simulink model "siasun_config_casadi_VS_lsj_sim_16a"  (R2019b)
settings: Solver=FixedStepAuto  StartTime=0.0  StopTime=20  FixedStep=0.001  RelTol=1e-3  EnableMultiTasking=on
undefined symbols (not defined in the file): a1, a2, a3, d1, d4, fc1, fc2, fc3, fc4, fc5, fc6, fv1, fv2, fv3, fv4, fv5, fv6, Ia1, Ia2, Ia3, Ia4, Ia5, Ia6, Ic111, Ic112, Ic113, Ic122, Ic123, Ic133, Ic211, Ic212, Ic213, Ic222, Ic223, Ic233, Ic311, Ic312, Ic313, Ic322, Ic323, Ic333, Ic411, Ic412, Ic413, Ic422, Ic423, Ic433, Ic511, Ic512, Ic513, Ic522, Ic523, Ic533, Ic611, Ic612, Ic613, Ic622, Ic623, Ic633, m1 ... (+26)
libraries: sm_lib x224, nesl_utility x124, simulink x8
(part 1 of 10)
settings Model: Creator=Administrator  LastModifiedBy=admin
settings SolverCC: AlgebraicLoopSolver=LineSearch
settings DataIOCC: ReturnWorkspaceOutputs=off
settings OptimizationCC: LifeSpan=inf
settings DebuggingCC: SFUnexpectedBacktrackingDiag=warning  SFNoUnconditionalDefaultTransitionDiag=warning  ArithmeticOperatorsInVariantConditions=warning
settings SFSimCC: SimUseLocalCustomCode=off  CustomCodeUndefinedFunction=UseInterfaceOnly
settings RTWCC: RTWUseLocalCustomCode=off
settings CodeAppCC: StateflowObjectComments=on
settings GRTTargetCC: TargetLangStandard=C89/C90 (ANSI)
settings ConfigComp: CovMetricSettings=dw  CovSaveCumulativeToWorkspaceVar=on  CovSaveSingleToWorkspaceVar=on  CovExternalEMLEnable=off
settings SimscapeCC: SimscapeNormalizeSystem=off
settings ExplorerConfigSet: InternalSimMechanicsExplorerSettings="<ExplorerConfiguration><canonicalview>default</canonicalview><AnimationSetting><BasePlaybackSpeed>1.0</BasePlaybackSpeed><PlaybackSpeedFactor>1.0</PlaybackSpeedFactor></AnimationSetting><TilePanel><TileInfo><Tiles Columns=\"1\" Count=\"1\" Rows=\"1\"><Column Left=\"2\" Weight=\"1\"/><Column Left=\"307\"/><Row Top=\"2\" Weight=\"1\"/><Row Top=\"464\"/><Tile Height=\"1\" Width=\"1\" X=\"0\" Y=\"0\"/></Tiles></TileInfo><SceneInfo><SceneViewer><BGColor><R>0.60000002384185791</R><G>0.60000002384185791</G><B>0.60000002384185791</B></BGColor><Camera><DoPerspective>off</DoPerspective><Position><X>0.25771122604707614</X><Y>-0.76959052816919193</Y><Z>0.37589669226781303</Z></Position><Center><X>0.25771122604707614</X><Y>0.14257423281669612</Y><Z>0.37589669226781303</Z></Center><Up><X>0</X><Y>-0</Y><Z>1</Z></Up><ViewLimDist>1</ViewLimDist><YLim>0.6801680654881832</YLim><XLim>0.44443652844260978</XLim></Camera></SceneViewer></SceneInfo></TilePanel><MechEditorPanel><Cameras/><GfxPanelCameraMap/></MechEditorPanel></ExplorerConfiguration>"

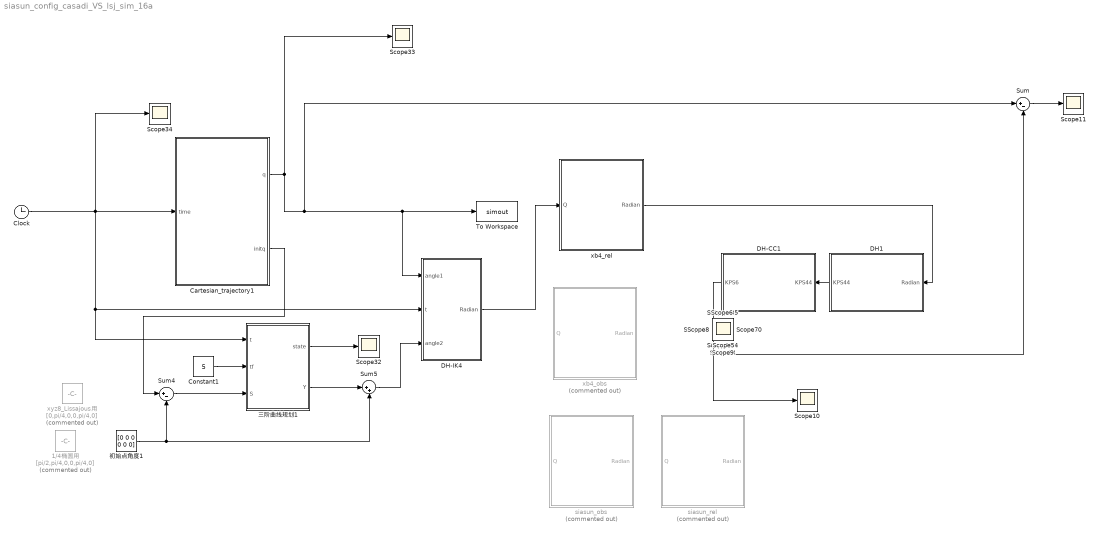
== system siasun_config_casadi_VS_lsj_sim_16a ==
  1/4椭圆用 : Constant  Commented=on  Value=[pi/2,pi/4,0,0,pi/4,0]
  Cartesian_trajectory1 : MATLAB Function  TreatAsAtomicUnit=on
  Clock : Clock
  Constant1 : Constant  Value=5
  DH-CC1 : MATLAB Function  TreatAsAtomicUnit=on
  DH-IK4 : MATLAB Function  TreatAsAtomicUnit=on
  DH1 : MATLAB Function  TreatAsAtomicUnit=on
  Scope{,1..34} (35 alike) : Scope
  Sum : Sum  Inputs=|+-
  Sum4 : Sum  Inputs=|+-
  Sum5 : Sum  Inputs=|++
  To Workspace : ToWorkspace  VariableName=simout  SampleTime=-1
      settings: Save2DSignal=2-D array (concatenate along first dimension)
  siasun_obs : Subsystem  Commented=on
  siasun_rel : Subsystem  Commented=on
  xb4_obs : Subsystem  Commented=on
  xb4_rel : Subsystem
  xyz8_Lissajous用 : Constant  Commented=on  Value=[0,pi/4,0,0,pi/4,0]
  三阶曲线规划1 : Subsystem
  初始点角度1 : Constant  Value=[0 0 0 0 0 0]
  wires:
  DH-IK4/1(Radian) -> xb4_rel/1(Q)
  Cartesian_trajectory1/1(q) -> To Workspace/1, DH-IK4/1(angle1), Sum/1, Scope33/1
  初始点角度1/1 -> Sum5/2, Sum4/2
  Sum4/1 -> 三阶曲线规划1/3(S)
  Constant1/1 -> 三阶曲线规划1/2(tf)
  三阶曲线规划1/1(state) -> Scope32/1
  三阶曲线规划1/2(Y) -> Sum5/1
  Sum5/1 -> DH-IK4/3(angle2)
  Clock/1 -> DH-IK4/2(t), 三阶曲线规划1/1(t), Scope34/1, Cartesian_trajectory1/1(time)
  xb4_rel/1(Radian) -> DH1/1(Radian)
  DH1/1(KPS44) -> DH-CC1/1(KPS44)
  DH-CC1/1(KPS6) -> Sum/2, Scope10/1
  Cartesian_trajectory1/2(initq) -> Sum4/1
  Sum/1 -> Scope11/1

== system siasun_config_casadi_VS_lsj_sim_16a/siasun_obs ==
  Q : Inport
  Discrete Derivative : simulink/Discrete/Discrete Derivative  gainval=1.0  ICPrevScaledInput=0.0  OutMin=[]  OutMax=[]  OutDataType=fixdt(1, 16)  OutScaling=2^-10  DoSatur=off
  Discrete Derivative1 : simulink/Discrete/Discrete Derivative  gainval=1.0  ICPrevScaledInput=0.0  OutMin=[]  OutMax=[]  OutDataType=fixdt(1, 16)  OutScaling=2^-10  DoSatur=off
  Robot : Subsystem
  Scope : Scope
  Scope1 : Scope
  Terminator : Terminator
  Terminator1 : Terminator
  Terminator2 : Terminator
  Radian : Outport
  wires:
  Discrete Derivative1/1 -> Robot/3(qdd), Scope/1
  Discrete Derivative/1 -> Robot/2(qd), Discrete Derivative1/1, Scope1/1
  Q/1 -> Robot/1(q), Discrete Derivative/1
  Robot/4(t) -> Terminator2/1
  Robot/3(b) -> Terminator1/1
  Robot/2(w) -> Terminator/1
  Robot/1(Q) -> Radian/1

== system siasun_config_casadi_VS_lsj_sim_16a/siasun_rel ==
  Q : Inport
  Discrete Derivative : simulink/Discrete/Discrete Derivative  gainval=1.0  ICPrevScaledInput=0.0  OutMin=[]  OutMax=[]  OutDataType=fixdt(1, 16)  OutScaling=2^-10  DoSatur=off
  Discrete Derivative1 : simulink/Discrete/Discrete Derivative  gainval=1.0  ICPrevScaledInput=0.0  OutMin=[]  OutMax=[]  OutDataType=fixdt(1, 16)  OutScaling=2^-10  DoSatur=off
  Robot : Subsystem
  Scope : Scope
  Scope1 : Scope
  Terminator : Terminator
  Terminator1 : Terminator
  Terminator2 : Terminator
  Radian : Outport
  wires:
  Discrete Derivative1/1 -> Robot/3(qdd), Scope/1
  Discrete Derivative/1 -> Robot/2(qd), Discrete Derivative1/1, Scope1/1
  Q/1 -> Robot/1(q), Discrete Derivative/1
  Robot/4(t) -> Terminator2/1
  Robot/3(b) -> Terminator1/1
  Robot/2(w) -> Terminator/1
  Robot/1(Q) -> Radian/1

== system siasun_config_casadi_VS_lsj_sim_16a/xb4_obs ==
  Q : Inport
  Discrete Derivative : simulink/Discrete/Discrete Derivative  gainval=1.0  ICPrevScaledInput=0.0  OutMin=[]  OutMax=[]  OutDataType=fixdt(1, 16)  OutScaling=2^-10  DoSatur=off
  Discrete Derivative1 : simulink/Discrete/Discrete Derivative  gainval=1.0  ICPrevScaledInput=0.0  OutMin=[]  OutMax=[]  OutDataType=fixdt(1, 16)  OutScaling=2^-10  DoSatur=off
  Robot : Subsystem
  Scope : Scope
  Scope1 : Scope
  Terminator : Terminator
  Terminator1 : Terminator
  Terminator2 : Terminator
  Radian : Outport
  wires:
  Discrete Derivative1/1 -> Robot/3(qdd), Scope/1
  Discrete Derivative/1 -> Robot/2(qd), Discrete Derivative1/1, Scope1/1
  Q/1 -> Robot/1(q), Discrete Derivative/1
  Robot/4(t) -> Terminator2/1
  Robot/3(b) -> Terminator1/1
  Robot/2(w) -> Terminator/1
  Robot/1(Q) -> Radian/1

== system siasun_config_casadi_VS_lsj_sim_16a/xb4_rel ==
  Q : Inport
  Discrete Derivative : simulink/Discrete/Discrete Derivative  gainval=1.0  ICPrevScaledInput=0.0  OutMin=[]  OutMax=[]  OutDataType=fixdt(1, 16)  OutScaling=2^-10  DoSatur=off
  Discrete Derivative1 : simulink/Discrete/Discrete Derivative  gainval=1.0  ICPrevScaledInput=0.0  OutMin=[]  OutMax=[]  OutDataType=fixdt(1, 16)  OutScaling=2^-10  DoSatur=off
  Robot : Subsystem
  Scope : Scope
  Scope1 : Scope
  Terminator : Terminator
  Terminator1 : Terminator
  Terminator2 : Terminator
  Radian : Outport
  wires:
  Robot/1(Q) -> Radian/1
  Robot/2(w) -> Terminator/1
  Robot/3(b) -> Terminator1/1
  Robot/4(t) -> Terminator2/1
  Q/1 -> Discrete Derivative/1, Robot/1(q)
  Discrete Derivative/1 -> Scope1/1, Discrete Derivative1/1, Robot/2(qd)
  Discrete Derivative1/1 -> Scope/1, Robot/3(qdd)

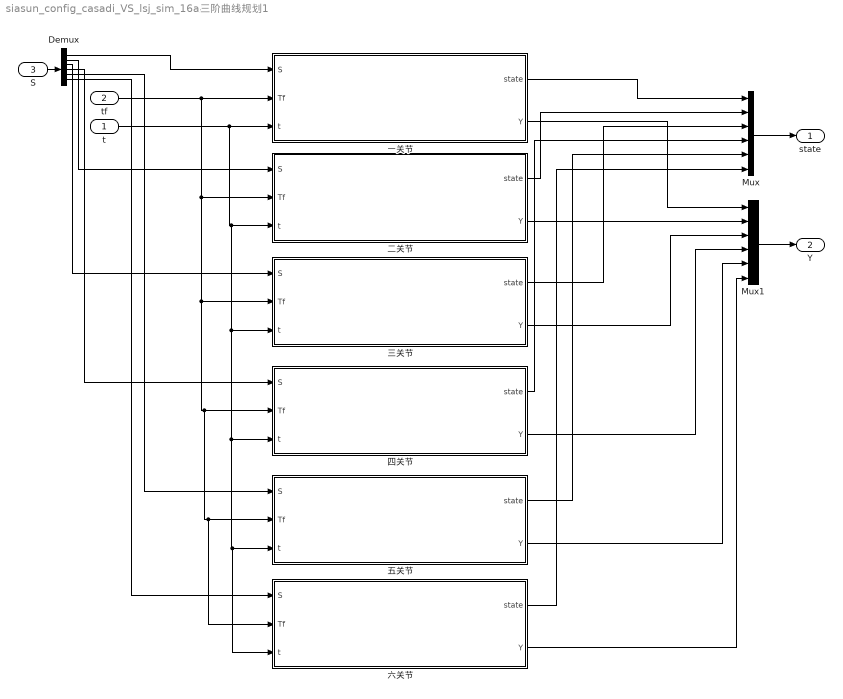
== system siasun_config_casadi_VS_lsj_sim_16a/三阶曲线规划1 ==
  t : Inport
  tf : Inport  Port=2
  S : Inport  Port=3
  Demux : Demux  Outputs=6
  Mux : Mux  Inputs=6
  Mux1 : Mux  Inputs=6
  一关节 : Subsystem
  三关节 : Subsystem
  二关节 : Subsystem
  五关节 : Subsystem
  六关节 : Subsystem
  四关节 : Subsystem
  state : Outport
  Y : Outport  Port=2
  wires:
  一关节/2(Y) -> Mux1/1
  tf/1 -> 六关节/2(Tf), 五关节/2(Tf), 四关节/2(Tf), 三关节/2(Tf), 二关节/2(Tf), 一关节/2(Tf)
  t/1 -> 六关节/3(t), 五关节/3(t), 四关节/3(t), 三关节/3(t), 二关节/3(t), 一关节/3(t)
  一关节/1(state) -> Mux/1
  三关节/1(state) -> Mux/3
  二关节/1(state) -> Mux/2
  四关节/1(state) -> Mux/4
  S/1 -> Demux/1
  Demux/1 -> 一关节/1(S)
  Demux/2 -> 二关节/1(S)
  Demux/3 -> 三关节/1(S)
  Demux/4 -> 四关节/1(S)
  Demux/5 -> 五关节/1(S)
  Demux/6 -> 六关节/1(S)
  Mux1/1 -> Y/1
  二关节/2(Y) -> Mux1/2
  三关节/2(Y) -> Mux1/3
  四关节/2(Y) -> Mux1/4
  五关节/2(Y) -> Mux1/5
  六关节/2(Y) -> Mux1/6
  Mux/1 -> state/1
  五关节/1(state) -> Mux/5
  六关节/1(state) -> Mux/6

== system siasun_config_casadi_VS_lsj_sim_16a/siasun_obs/Robot ==
  q : Inport
  qd : Inport  Port=2
  qdd : Inport  Port=3
  Robot : Subsystem
  Q : Outport
  w : Outport  Port=2
  b : Outport  Port=3
  t : Outport  Port=4
  wires:
  qdd/1 -> Robot/3(qdd)
  qd/1 -> Robot/2(qd)
  q/1 -> Robot/1(q)
  Robot/4(t) -> t/1
  Robot/3(b) -> b/1
  Robot/2(w) -> w/1
  Robot/1(Q) -> Q/1

== system siasun_config_casadi_VS_lsj_sim_16a/siasun_rel/Robot ==
  q : Inport
  qd : Inport  Port=2
  qdd : Inport  Port=3
  Robot : Subsystem
  Q : Outport
  w : Outport  Port=2
  b : Outport  Port=3
  t : Outport  Port=4
  wires:
  qdd/1 -> Robot/3(qdd)
  qd/1 -> Robot/2(qd)
  q/1 -> Robot/1(q)
  Robot/4(t) -> t/1
  Robot/3(b) -> b/1
  Robot/2(w) -> w/1
  Robot/1(Q) -> Q/1

== system siasun_config_casadi_VS_lsj_sim_16a/xb4_obs/Robot ==
  q : Inport
  qd : Inport  Port=2
  qdd : Inport  Port=3
  Robot : Subsystem
  Q : Outport
  w : Outport  Port=2
  b : Outport  Port=3
  t : Outport  Port=4
  wires:
  qdd/1 -> Robot/3(qdd)
  qd/1 -> Robot/2(qd)
  q/1 -> Robot/1(q)
  Robot/4(t) -> t/1
  Robot/3(b) -> b/1
  Robot/2(w) -> w/1
  Robot/1(Q) -> Q/1

== system siasun_config_casadi_VS_lsj_sim_16a/xb4_rel/Robot ==
  q : Inport
  qd : Inport  Port=2
  qdd : Inport  Port=3
  Robot : Subsystem
  Q : Outport
  w : Outport  Port=2
  b : Outport  Port=3
  t : Outport  Port=4
  wires:
  Robot/1(Q) -> Q/1
  Robot/2(w) -> w/1
  Robot/3(b) -> b/1
  Robot/4(t) -> t/1
  q/1 -> Robot/1(q)
  qd/1 -> Robot/2(qd)
  qdd/1 -> Robot/3(qdd)

== system siasun_config_casadi_VS_lsj_sim_16a/三阶曲线规划1/一关节 ==
  S : Inport
  Tf : Inport  Port=2
  t : Inport  Port=3
  3_planning1 : MATLAB Function  TreatAsAtomicUnit=on  mask{g_vs=0, g_ve=0}
      mask prompts: g_vs "初始速度"; g_ve "末速度"
  Interpolation3 : MATLAB Function  TreatAsAtomicUnit=on
  state : Outport
  Y : Outport  Port=2
  wires:
  t/1 -> Interpolation3/4(t)
  S/1 -> 3_planning1/1(S)
  3_planning1/1(state) -> Interpolation3/1(Enable)
  3_planning1/2(plan3_A) -> Interpolation3/2(plan3_A)
  3_planning1/3(tf) -> Interpolation3/3(tf)
  Tf/1 -> 3_planning1/2("tf ")
  Interpolation3/2(Y) -> Y/1
  Interpolation3/1(state) -> state/1

== system siasun_config_casadi_VS_lsj_sim_16a/三阶曲线规划1/三关节 ==
  S : Inport
  Tf : Inport  Port=2
  t : Inport  Port=3
  3_planning1 : MATLAB Function  TreatAsAtomicUnit=on  mask{g_vs=0, g_ve=0}
      mask prompts: g_vs "初始速度"; g_ve "末速度"
  Interpolation3 : MATLAB Function  TreatAsAtomicUnit=on
  state : Outport
  Y : Outport  Port=2
  wires:
  t/1 -> Interpolation3/4(t)
  S/1 -> 3_planning1/1(S)
  3_planning1/1(state) -> Interpolation3/1(Enable)
  3_planning1/2(plan3_A) -> Interpolation3/2(plan3_A)
  3_planning1/3(tf) -> Interpolation3/3(tf)
  Tf/1 -> 3_planning1/2("tf ")
  Interpolation3/2(Y) -> Y/1
  Interpolation3/1(state) -> state/1

== system siasun_config_casadi_VS_lsj_sim_16a/三阶曲线规划1/二关节 ==
  S : Inport
  Tf : Inport  Port=2
  t : Inport  Port=3
  3_planning1 : MATLAB Function  TreatAsAtomicUnit=on  mask{g_vs=0, g_ve=0}
      mask prompts: g_vs "初始速度"; g_ve "末速度"
  Interpolation3 : MATLAB Function  TreatAsAtomicUnit=on
  state : Outport
  Y : Outport  Port=2
  wires:
  t/1 -> Interpolation3/4(t)
  S/1 -> 3_planning1/1(S)
  3_planning1/1(state) -> Interpolation3/1(Enable)
  3_planning1/2(plan3_A) -> Interpolation3/2(plan3_A)
  3_planning1/3(tf) -> Interpolation3/3(tf)
  Tf/1 -> 3_planning1/2("tf ")
  Interpolation3/2(Y) -> Y/1
  Interpolation3/1(state) -> state/1

== system siasun_config_casadi_VS_lsj_sim_16a/三阶曲线规划1/五关节 ==
  S : Inport
  Tf : Inport  Port=2
  t : Inport  Port=3
  3_planning1 : MATLAB Function  TreatAsAtomicUnit=on  mask{g_vs=0, g_ve=0}
      mask prompts: g_vs "初始速度"; g_ve "末速度"
  Interpolation3 : MATLAB Function  TreatAsAtomicUnit=on
  state : Outport
  Y : Outport  Port=2
  wires:
  t/1 -> Interpolation3/4(t)
  S/1 -> 3_planning1/1(S)
  3_planning1/1(state) -> Interpolation3/1(Enable)
  3_planning1/2(plan3_A) -> Interpolation3/2(plan3_A)
  3_planning1/3(tf) -> Interpolation3/3(tf)
  Tf/1 -> 3_planning1/2("tf ")
  Interpolation3/2(Y) -> Y/1
  Interpolation3/1(state) -> state/1

== system siasun_config_casadi_VS_lsj_sim_16a/三阶曲线规划1/六关节 ==
  S : Inport
  Tf : Inport  Port=2
  t : Inport  Port=3
  3_planning1 : MATLAB Function  TreatAsAtomicUnit=on  mask{g_vs=0, g_ve=0}
      mask prompts: g_vs "初始速度"; g_ve "末速度"
  Interpolation3 : MATLAB Function  TreatAsAtomicUnit=on
  state : Outport
  Y : Outport  Port=2
  wires:
  t/1 -> Interpolation3/4(t)
  S/1 -> 3_planning1/1(S)
  3_planning1/1(state) -> Interpolation3/1(Enable)
  3_planning1/2(plan3_A) -> Interpolation3/2(plan3_A)
  3_planning1/3(tf) -> Interpolation3/3(tf)
  Tf/1 -> 3_planning1/2("tf ")
  Interpolation3/2(Y) -> Y/1
  Interpolation3/1(state) -> state/1

== system siasun_config_casadi_VS_lsj_sim_16a/三阶曲线规划1/四关节 ==
  S : Inport
  Tf : Inport  Port=2
  t : Inport  Port=3
  3_planning1 : MATLAB Function  TreatAsAtomicUnit=on  mask{g_vs=0, g_ve=0}
      mask prompts: g_vs "初始速度"; g_ve "末速度"
  Interpolation3 : MATLAB Function  TreatAsAtomicUnit=on
  state : Outport
  Y : Outport  Port=2
  wires:
  t/1 -> Interpolation3/4(t)
  S/1 -> 3_planning1/1(S)
  3_planning1/1(state) -> Interpolation3/1(Enable)
  3_planning1/2(plan3_A) -> Interpolation3/2(plan3_A)
  3_planning1/3(tf) -> Interpolation3/3(tf)
  Tf/1 -> 3_planning1/2("tf ")
  Interpolation3/2(Y) -> Y/1
  Interpolation3/1(state) -> state/1

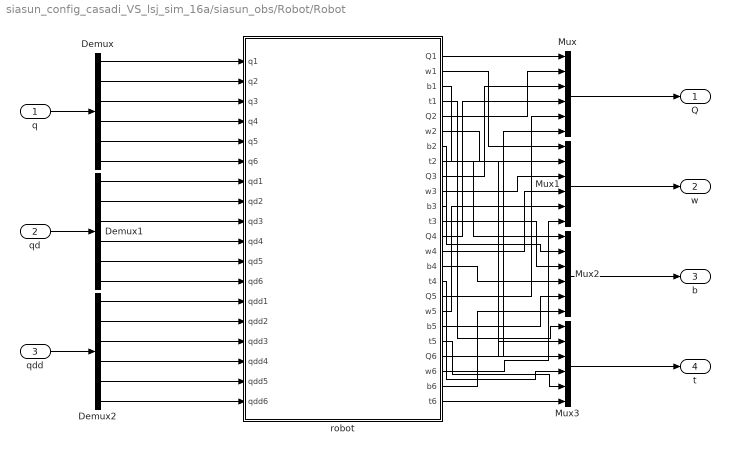
== system siasun_config_casadi_VS_lsj_sim_16a/siasun_obs/Robot/Robot ==
  q : Inport
  qd : Inport  Port=2
  qdd : Inport  Port=3
  Demux : Demux  Outputs=6
  Demux1 : Demux  Outputs=6
  Demux2 : Demux  Outputs=6
  Mux{,1..3} (4 alike) : Mux  Inputs=6
  robot : Subsystem
  Q : Outport
  w : Outport  Port=2
  b : Outport  Port=3
  t : Outport  Port=4
  wires:
  qdd/1 -> Demux2/1
  Demux2/1 -> robot/13(qdd1)
  Demux2/6 -> robot/18(qdd6)
  Demux2/5 -> robot/17(qdd5)
  Demux2/4 -> robot/16(qdd4)
  Demux2/3 -> robot/15(qdd3)
  Demux2/2 -> robot/14(qdd2)
  qd/1 -> Demux1/1
  Demux1/1 -> robot/7(qd1)
  Demux1/6 -> robot/12(qd6)
  Demux1/5 -> robot/11(qd5)
  Demux1/4 -> robot/10(qd4)
  Demux1/3 -> robot/9(qd3)
  Demux1/2 -> robot/8(qd2)
  Demux/6 -> robot/6(q6)
  Demux/5 -> robot/5(q5)
  Demux/4 -> robot/4(q4)
  Demux/3 -> robot/3(q3)
  Demux/2 -> robot/2(q2)
  Demux/1 -> robot/1(q1)
  Mux3/1 -> t/1
  Mux2/1 -> b/1
  Mux1/1 -> w/1
  Mux/1 -> Q/1
  robot/24(t6) -> Mux3/6
  robot/20(t5) -> Mux3/5
  robot/16(t4) -> Mux3/4
  robot/12(t3) -> Mux3/3
  robot/8(t2) -> Mux3/2
  robot/4(t1) -> Mux3/1
  robot/23(b6) -> Mux2/6
  robot/19(b5) -> Mux2/5
  robot/15(b4) -> Mux2/4
  robot/11(b3) -> Mux2/3
  robot/7(b2) -> Mux2/2
  robot/22(w6) -> Mux1/6
  robot/18(w5) -> Mux1/5
  robot/14(w4) -> Mux1/4
  robot/10(w3) -> Mux1/3
  robot/6(w2) -> Mux1/2
  robot/3(b1) -> Mux2/1
  robot/2(w1) -> Mux1/1
  robot/21(Q6) -> Mux/6
  robot/17(Q5) -> Mux/5
  robot/13(Q4) -> Mux/4
  robot/9(Q3) -> Mux/3
  robot/5(Q2) -> Mux/2
  robot/1(Q1) -> Mux/1
  q/1 -> Demux/1

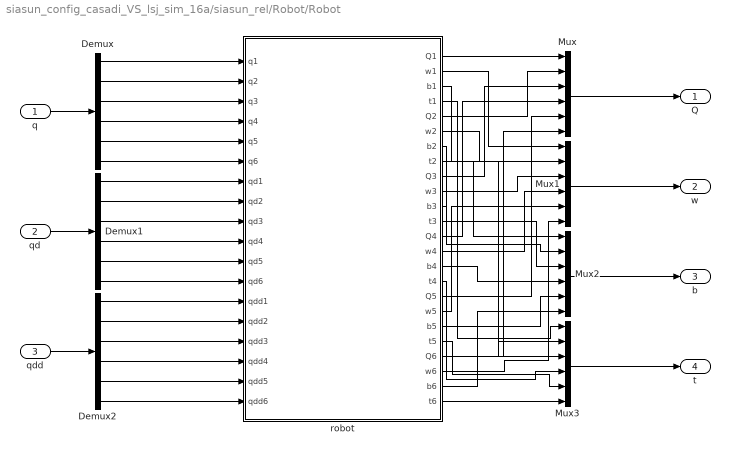
== system siasun_config_casadi_VS_lsj_sim_16a/siasun_rel/Robot/Robot ==
  q : Inport
  qd : Inport  Port=2
  qdd : Inport  Port=3
  Demux : Demux  Outputs=6
  Demux1 : Demux  Outputs=6
  Demux2 : Demux  Outputs=6
  Mux{,1..3} (4 alike) : Mux  Inputs=6
  robot : Subsystem
  Q : Outport
  w : Outport  Port=2
  b : Outport  Port=3
  t : Outport  Port=4
  wires:
  qdd/1 -> Demux2/1
  Demux2/1 -> robot/13(qdd1)
  Demux2/6 -> robot/18(qdd6)
  Demux2/5 -> robot/17(qdd5)
  Demux2/4 -> robot/16(qdd4)
  Demux2/3 -> robot/15(qdd3)
  Demux2/2 -> robot/14(qdd2)
  qd/1 -> Demux1/1
  Demux1/1 -> robot/7(qd1)
  Demux1/6 -> robot/12(qd6)
  Demux1/5 -> robot/11(qd5)
  Demux1/4 -> robot/10(qd4)
  Demux1/3 -> robot/9(qd3)
  Demux1/2 -> robot/8(qd2)
  Demux/6 -> robot/6(q6)
  Demux/5 -> robot/5(q5)
  Demux/4 -> robot/4(q4)
  Demux/3 -> robot/3(q3)
  Demux/2 -> robot/2(q2)
  Demux/1 -> robot/1(q1)
  Mux3/1 -> t/1
  Mux2/1 -> b/1
  Mux1/1 -> w/1
  Mux/1 -> Q/1
  robot/24(t6) -> Mux3/6
  robot/20(t5) -> Mux3/5
  robot/16(t4) -> Mux3/4
  robot/12(t3) -> Mux3/3
  robot/8(t2) -> Mux3/2
  robot/4(t1) -> Mux3/1
  robot/23(b6) -> Mux2/6
  robot/19(b5) -> Mux2/5
  robot/15(b4) -> Mux2/4
  robot/11(b3) -> Mux2/3
  robot/7(b2) -> Mux2/2
  robot/22(w6) -> Mux1/6
  robot/18(w5) -> Mux1/5
  robot/14(w4) -> Mux1/4
  robot/10(w3) -> Mux1/3
  robot/6(w2) -> Mux1/2
  robot/3(b1) -> Mux2/1
  robot/2(w1) -> Mux1/1
  robot/21(Q6) -> Mux/6
  robot/17(Q5) -> Mux/5
  robot/13(Q4) -> Mux/4
  robot/9(Q3) -> Mux/3
  robot/5(Q2) -> Mux/2
  robot/1(Q1) -> Mux/1
  q/1 -> Demux/1

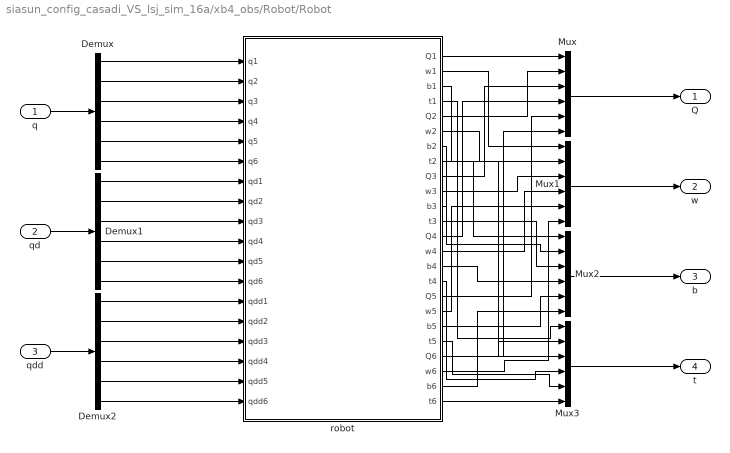
== system siasun_config_casadi_VS_lsj_sim_16a/xb4_obs/Robot/Robot ==
  q : Inport
  qd : Inport  Port=2
  qdd : Inport  Port=3
  Demux : Demux  Outputs=6
  Demux1 : Demux  Outputs=6
  Demux2 : Demux  Outputs=6
  Mux{,1..3} (4 alike) : Mux  Inputs=6
  robot : Subsystem
  Q : Outport
  w : Outport  Port=2
  b : Outport  Port=3
  t : Outport  Port=4
  wires:
  qdd/1 -> Demux2/1
  Demux2/1 -> robot/13(qdd1)
  Demux2/6 -> robot/18(qdd6)
  Demux2/5 -> robot/17(qdd5)
  Demux2/4 -> robot/16(qdd4)
  Demux2/3 -> robot/15(qdd3)
  Demux2/2 -> robot/14(qdd2)
  qd/1 -> Demux1/1
  Demux1/1 -> robot/7(qd1)
  Demux1/6 -> robot/12(qd6)
  Demux1/5 -> robot/11(qd5)
  Demux1/4 -> robot/10(qd4)
  Demux1/3 -> robot/9(qd3)
  Demux1/2 -> robot/8(qd2)
  Demux/6 -> robot/6(q6)
  Demux/5 -> robot/5(q5)
  Demux/4 -> robot/4(q4)
  Demux/3 -> robot/3(q3)
  Demux/2 -> robot/2(q2)
  Demux/1 -> robot/1(q1)
  Mux3/1 -> t/1
  Mux2/1 -> b/1
  Mux1/1 -> w/1
  Mux/1 -> Q/1
  robot/24(t6) -> Mux3/6
  robot/20(t5) -> Mux3/5
  robot/16(t4) -> Mux3/4
  robot/12(t3) -> Mux3/3
  robot/8(t2) -> Mux3/2
  robot/4(t1) -> Mux3/1
  robot/23(b6) -> Mux2/6
  robot/19(b5) -> Mux2/5
  robot/15(b4) -> Mux2/4
  robot/11(b3) -> Mux2/3
  robot/7(b2) -> Mux2/2
  robot/22(w6) -> Mux1/6
  robot/18(w5) -> Mux1/5
  robot/14(w4) -> Mux1/4
  robot/10(w3) -> Mux1/3
  robot/6(w2) -> Mux1/2
  robot/3(b1) -> Mux2/1
  robot/2(w1) -> Mux1/1
  robot/21(Q6) -> Mux/6
  robot/17(Q5) -> Mux/5
  robot/13(Q4) -> Mux/4
  robot/9(Q3) -> Mux/3
  robot/5(Q2) -> Mux/2
  robot/1(Q1) -> Mux/1
  q/1 -> Demux/1

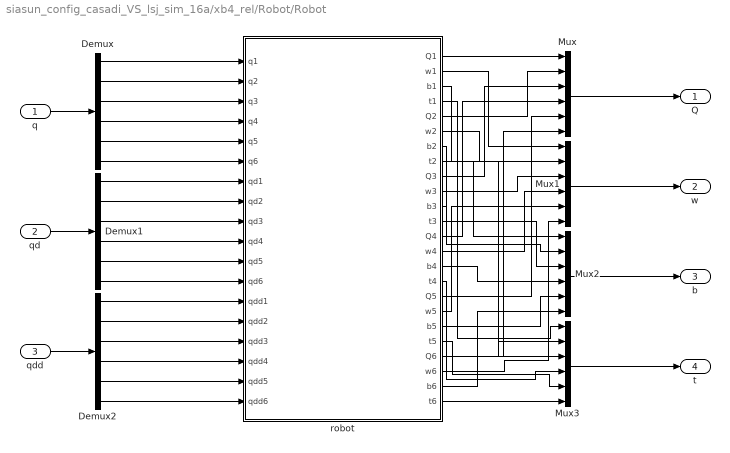
== system siasun_config_casadi_VS_lsj_sim_16a/xb4_rel/Robot/Robot ==
  q : Inport
  qd : Inport  Port=2
  qdd : Inport  Port=3
  Demux : Demux  Outputs=6
  Demux1 : Demux  Outputs=6
  Demux2 : Demux  Outputs=6
  Mux{,1..3} (4 alike) : Mux  Inputs=6
  robot : Subsystem
  Q : Outport
  w : Outport  Port=2
  b : Outport  Port=3
  t : Outport  Port=4
  wires:
  q/1 -> Demux/1
  robot/1(Q1) -> Mux/1
  robot/5(Q2) -> Mux/2
  robot/9(Q3) -> Mux/3
  robot/13(Q4) -> Mux/4
  robot/17(Q5) -> Mux/5
  robot/21(Q6) -> Mux/6
  robot/2(w1) -> Mux1/1
  robot/3(b1) -> Mux2/1
  robot/6(w2) -> Mux1/2
  robot/10(w3) -> Mux1/3
  robot/14(w4) -> Mux1/4
  robot/18(w5) -> Mux1/5
  robot/22(w6) -> Mux1/6
  robot/7(b2) -> Mux2/2
  robot/11(b3) -> Mux2/3
  robot/15(b4) -> Mux2/4
  robot/19(b5) -> Mux2/5
  robot/23(b6) -> Mux2/6
  robot/4(t1) -> Mux3/1
  robot/8(t2) -> Mux3/2
  robot/12(t3) -> Mux3/3
  robot/16(t4) -> Mux3/4
  robot/20(t5) -> Mux3/5
  robot/24(t6) -> Mux3/6
  Mux/1 -> Q/1
  Mux1/1 -> w/1
  Mux2/1 -> b/1
  Mux3/1 -> t/1
  Demux/1 -> robot/1(q1)
  Demux/2 -> robot/2(q2)
  Demux/3 -> robot/3(q3)
  Demux/4 -> robot/4(q4)
  Demux/5 -> robot/5(q5)
  Demux/6 -> robot/6(q6)
  Demux1/2 -> robot/8(qd2)
  Demux1/3 -> robot/9(qd3)
  Demux1/4 -> robot/10(qd4)
  Demux1/5 -> robot/11(qd5)
  Demux1/6 -> robot/12(qd6)
  Demux1/1 -> robot/7(qd1)
  qd/1 -> Demux1/1
  Demux2/2 -> robot/14(qdd2)
  Demux2/3 -> robot/15(qdd3)
  Demux2/4 -> robot/16(qdd4)
  Demux2/5 -> robot/17(qdd5)
  Demux2/6 -> robot/18(qdd6)
  Demux2/1 -> robot/13(qdd1)
  qdd/1 -> Demux2/1

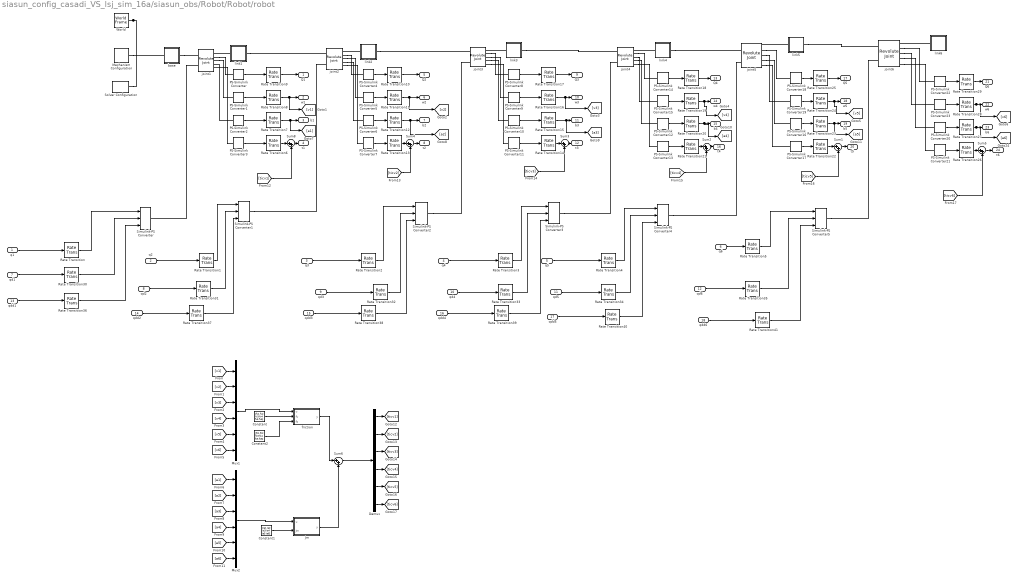
== system siasun_config_casadi_VS_lsj_sim_16a/siasun_obs/Robot/Robot/robot ==
  q1 : Inport
  q2 : Inport  Port=2
  q3 : Inport  Port=3
  q4 : Inport  Port=4
  q5 : Inport  Port=5
  q6 : Inport  Port=6
  qd1 : Inport  Port=7
  qd2 : Inport  Port=8
  qd3 : Inport  Port=9
  qd4 : Inport  Port=10
  qd5 : Inport  Port=11
  qd6 : Inport  Port=12
  qdd1 : Inport  Port=13
  qdd2 : Inport  Port=14
  qdd3 : Inport  Port=15
  qdd4 : Inport  Port=16
  qdd5 : Inport  Port=17
  qdd6 : Inport  Port=18
  Constant : Constant  Value=[fv1 fv2 fv3 fv4 fv5 fv6]
  Constant1 : Constant  Value=[Ia1 Ia2 Ia3 Ia4 Ia5 Ia6]
  Constant2 : Constant  Value=[fc1 fc2 fc3 fc4 fc5 fc6]
  Demux : Demux  Outputs=6
  Jm : MATLAB Function  TreatAsAtomicUnit=on
  Mechanism Configuration : sm_lib/Utilities/Mechanism Configuration  UniformGravity=Constant  GravityVector=[0 0 -9.802]  GravityUnits=m/s^2  LinearizationDelta=0.001
  Mux1 : Mux  Inputs=6
  Mux2 : Mux  Inputs=6
  PS-Simulink Converter{,4,8,14,18,22} (6 alike) : nesl_utility/PS-Simulink Converter  PhysicalDomain=network_engine_domain  SubClassName=ps_output  LeftPortType=input  RightPortType=output  PseudoPeriodic=off  Frequencies=[]  Unit=rad  AffineConversion=off
  PS-Simulink Converter{1,5,9,15,19,23} (6 alike) : nesl_utility/PS-Simulink Converter  PhysicalDomain=network_engine_domain  SubClassName=ps_output  LeftPortType=input  RightPortType=output  PseudoPeriodic=off  Frequencies=[]  Unit=rad/s  AffineConversion=off
  PS-Simulink Converter{2,6,10,12,16,20} (6 alike) : nesl_utility/PS-Simulink Converter  PhysicalDomain=network_engine_domain  SubClassName=ps_output  LeftPortType=input  RightPortType=output  PseudoPeriodic=off  Frequencies=[]  Unit=1  AffineConversion=off
  PS-Simulink Converter{3,7,11,13,17,21} (6 alike) : nesl_utility/PS-Simulink Converter  PhysicalDomain=network_engine_domain  SubClassName=ps_output  LeftPortType=input  RightPortType=output  PseudoPeriodic=off  Frequencies=[]  Unit=N*m  AffineConversion=off
  Rate Transition{,1..41} (42 alike) : RateTransition
  Simulink-PS Converter{,1..5} (6 alike) : nesl_utility/Simulink-PS Converter  PhysicalDomain=network_engine_domain  SubClassName=ps_input  LeftPortType=input  RightPortType=output  PseudoPeriodic=off  Frequencies=[]  NoiseDistribution=none  NoiseParameters=[]  Unit=rad  AffineConversion=off  FilteringAndDerivatives=provide  SimscapeFilterOrder=1  InputFilterTimeConstant=0.001  UdotUserProvided=2
  Solver Configuration : nesl_utility/Solver Configuration  PhysicalDomain=network_engine_domain  SubClassName=solver  LeftPortType=input  RightPortType=generic  Tones=[]  Harmonics=[]  SimulateNoise=off  Profile=off  UseLocalSampling=off  EnableSwitchedLinearOptims=on  FrequencyDomain=off  UseCCode=off  RelTol=0.001  AbsTol=1e-06  MinStep=1e-09  ToWorkspace=off  RevertToSquareIcSolve=off  NumHomotopyIterations=100  PhasorMode=off  PhasorModeNumHarmonics=1  DoDC=off  ResidualTolerance=1e-09  UseLocalSolver=off  LocalSolverChoice=NE_BACKWARD_EULER_ADVANCER  LocalSolverSampleTime=0.001  DoFixedCost=off  MaxNonlinIter=3  MaxModeIter=2  LinearAlgebra=Sparse  EquationFormulation=NE_TIME_EF  DelaysMemoryBudget=1024  AutomaticFiltering=on  FilteringTimeConstant=0.001  PartitionStorageMethod=AS_NEEDED  PartitionMemoryBudget=1024  PartitionMethod=FAST
  Sum{1..6,8} (7 alike) : Sum  Inputs=|++
  World : sm_lib/Frames and Transforms/World Frame
  base : Subsystem
  friction : MATLAB Function  TreatAsAtomicUnit=on
  joint1 : sm_lib/Joints/Revolute Joint  JointMode=Normal  SenseConstraintForce=off  SenseConstraintForceX=off  SenseConstraintForceY=off  SenseConstraintForceZ=off  SenseConstraintTorque=off  SenseConstraintTorqueX=off  SenseConstraintTorqueY=off  SenseConstraintTorqueZ=off  SenseTotalForce=off  SenseTotalForceX=off  SenseTotalForceY=off  SenseTotalForceZ=off  SenseTotalTorque=off  SenseTotalTorqueX=off  SenseTotalTorqueY=off  SenseTotalTorqueZ=off  CompositeWrenchDir=FollowerOnBase  CompositeWrenchFrame=FollowerFrame  EquilibriumPosition=0  EquilibriumPositionUnits=deg  SpringStiffness=0  SpringStiffnessUnits=N*m/deg  DampingCoefficient=0  DampingCoefficientUnits=N*m/(deg/s)  TorqueActuationMode=ComputedTorque  MotionActuationMode=InputMotion  SensePosition=on  SenseVelocity=on  SenseAcceleration=on  SenseTorqueForce=on  SenseLowerLimitTorqueForce=off  SenseUpperLimitTorqueForce=off  LowerLimitSpecify=off  LowerLimitBound=-90  LowerLimitBoundUnits=deg  LowerLimitStiffness=1e4  LowerLimitStiffnessUnits=N*m/deg  LowerLimitDamping=10  LowerLimitDampingUnits=N*m/(deg/s)  LowerLimitTransitionRegionWidth=0.1  LowerLimitTransitionRegionWidthUnits=deg  UpperLimitSpecify=off  UpperLimitBound=90  UpperLimitBoundUnits=deg  UpperLimitStiffness=1e4  UpperLimitStiffnessUnits=N*m/deg  UpperLimitDamping=10  UpperLimitDampingUnits=N*m/(deg/s)  UpperLimitTransitionRegionWidth=0.1  UpperLimitTransitionRegionWidthUnits=deg  PositionTargetSpecify=off  PositionTargetPriority=High  PositionTargetValue=0  PositionTargetValueUnits=deg  VelocityTargetSpecify=off  VelocityTargetPriority=High  VelocityTargetValue=0  VelocityTargetValueUnits=deg/s
  joint{2..6} (5 alike) : sm_lib/Joints/Revolute Joint  JointMode=Normal  SenseConstraintForce=off  SenseConstraintForceX=off  SenseConstraintForceY=off  SenseConstraintForceZ=off  SenseConstraintTorque=off  SenseConstraintTorqueX=off  SenseConstraintTorqueY=off  SenseConstraintTorqueZ=off  SenseTotalForce=off  SenseTotalForceX=off  SenseTotalForceY=off  SenseTotalForceZ=off  SenseTotalTorque=off  SenseTotalTorqueX=off  SenseTotalTorqueY=off  SenseTotalTorqueZ=off  CompositeWrenchDir=FollowerOnBase  CompositeWrenchFrame=BaseFrame  EquilibriumPosition=0  EquilibriumPositionUnits=deg  SpringStiffness=0  SpringStiffnessUnits=N*m/deg  DampingCoefficient=0  DampingCoefficientUnits=N*m/(deg/s)  TorqueActuationMode=ComputedTorque  MotionActuationMode=InputMotion  SensePosition=on  SenseVelocity=on  SenseAcceleration=on  SenseTorqueForce=on  SenseLowerLimitTorqueForce=off  SenseUpperLimitTorqueForce=off  LowerLimitSpecify=off  LowerLimitBound=-90  LowerLimitBoundUnits=deg  LowerLimitStiffness=1e4  LowerLimitStiffnessUnits=N*m/deg  LowerLimitDamping=10  LowerLimitDampingUnits=N*m/(deg/s)  LowerLimitTransitionRegionWidth=0.1  LowerLimitTransitionRegionWidthUnits=deg  UpperLimitSpecify=off  UpperLimitBound=90  UpperLimitBoundUnits=deg  UpperLimitStiffness=1e4  UpperLimitStiffnessUnits=N*m/deg  UpperLimitDamping=10  UpperLimitDampingUnits=N*m/(deg/s)  UpperLimitTransitionRegionWidth=0.1  UpperLimitTransitionRegionWidthUnits=deg  PositionTargetSpecify=off  PositionTargetPriority=High  PositionTargetValue=0  PositionTargetValueUnits=deg  VelocityTargetSpecify=off  VelocityTargetPriority=High  VelocityTargetValue=0  VelocityTargetValueUnits=deg/s
  link1 : Subsystem
  link2 : Subsystem
  link3 : Subsystem
  link4 : Subsystem
  link5 : Subsystem
  link6 : Subsystem
  Q1 : Outport
  w1 : Outport  Port=2
  b1 : Outport  Port=3
  t1 : Outport  Port=4
  Q2 : Outport  Port=5
  w2 : Outport  Port=6
  b2 : Outport  Port=7
  t2 : Outport  Port=8
  Q3 : Outport  Port=9
  w3 : Outport  Port=10
  b3 : Outport  Port=11
  t3 : Outport  Port=12
  Q4 : Outport  Port=13
  w4 : Outport  Port=14
  b4 : Outport  Port=15
  t4 : Outport  Port=16
  Q5 : Outport  Port=17
  w5 : Outport  Port=18
  b5 : Outport  Port=19
  t5 : Outport  Port=20
  Q6 : Outport  Port=21
  w6 : Outport  Port=22
  b6 : Outport  Port=23
  t6 : Outport  Port=24
  wires:
  Rate Transition41/1 -> Simulink-PS Converter5/3
  qdd6/1 -> Rate Transition41/1
  Rate Transition40/1 -> Simulink-PS Converter4/3
  qdd5/1 -> Rate Transition40/1
  Rate Transition39/1 -> Simulink-PS Converter3/3
  qdd4/1 -> Rate Transition39/1
  Rate Transition38/1 -> Simulink-PS Converter2/3
  qdd3/1 -> Rate Transition38/1
  Rate Transition37/1 -> Simulink-PS Converter1/3
  qdd2/1 -> Rate Transition37/1
  Rate Transition36/1 -> Simulink-PS Converter/3
  qdd1/1 -> Rate Transition36/1
  Rate Transition35/1 -> Simulink-PS Converter5/2
  qd6/1 -> Rate Transition35/1
  Rate Transition34/1 -> Simulink-PS Converter4/2
  qd5/1 -> Rate Transition34/1
  Rate Transition33/1 -> Simulink-PS Converter3/2
  qd4/1 -> Rate Transition33/1
  Rate Transition32/1 -> Simulink-PS Converter2/2
  qd3/1 -> Rate Transition32/1
  Rate Transition31/1 -> Simulink-PS Converter1/2
  qd2/1 -> Rate Transition31/1
  Rate Transition30/1 -> Simulink-PS Converter/2
  qd1/1 -> Rate Transition30/1
  Rate Transition6/1 -> Sum8/1
  Sum8/1 -> t1/1
  [ticv2] -> Sum4/2
  Sum4/1 -> t2/1
  Rate Transition13/1 -> Sum4/1
  Sum3/1 -> t3/1
  Rate Transition14/1 -> Sum3/1
  Sum2/1 -> t4/1
  Rate Transition21/1 -> Sum2/1
  Sum1/1 -> t5/1
  Rate Transition22/1 -> Sum1/1
  Sum5/1 -> t6/1
  Rate Transition26/1 -> Sum5/1
  q6/1 -> Rate Transition5/1
  q5/1 -> Rate Transition4/1
  q4/1 -> Rate Transition3/1
  q3/1 -> Rate Transition2/1
  q2/1 -> Rate Transition1/1
  q1/1 -> Rate Transition/1
  Sum6/1 -> Demux/1
  Constant2/1 -> friction/3(fc)
  Constant1/1 -> Jm/2(Jm)
  Constant/1 -> friction/2(fv)
  Jm/1(y) -> Sum6/2
  friction/1(y) -> Sum6/1
  Mux2/1 -> Jm/1(u)
  Mux1/1 -> friction/1(u)
  [ticv6] -> Sum5/2
  [ticv5] -> Sum1/2
  [ticv4] -> Sum2/2
  [ticv3] -> Sum3/2
  [ticv1] -> Sum8/2
  Demux/6 -> [ticv6]
  Demux/5 -> [ticv5]
  Demux/4 -> [ticv4]
  Demux/3 -> [ticv3]
  Demux/2 -> [ticv2]
  Demux/1 -> [ticv1]
  [a6] -> Mux2/6
  [a4] -> Mux2/4
  [a5] -> Mux2/5
  [a3] -> Mux2/3
  [a2] -> Mux2/2
  [a1] -> Mux2/1
  [v6] -> Mux1/6
  [v5] -> Mux1/5
  [v4] -> Mux1/4
  [v3] -> Mux1/3
  [v2] -> Mux1/2
  [v1] -> Mux1/1
  Rate Transition29/1 -> Q6/1
  Rate Transition28/1 -> w6/1, [v6]
  Rate Transition27/1 -> b6/1, [a6]
  Rate Transition25/1 -> Q5/1
  Rate Transition24/1 -> w5/1, [v5]
  Rate Transition23/1 -> b5/1, [a5]
  Rate Transition20/1 -> b4/1, [a4]
  Rate Transition19/1 -> w4/1, [v4]
  Rate Transition18/1 -> Q4/1
  Rate Transition17/1 -> Q3/1
  Rate Transition16/1 -> w3/1, [v3]
  Rate Transition15/1 -> b3/1, [a3]
  Rate Transition12/1 -> b2/1, [a2]
  Rate Transition11/1 -> w2/1, [v2]
  Rate Transition10/1 -> Q2/1
  Rate Transition9/1 -> Q1/1
  Rate Transition8/1 -> w1/1, [v1]
  Rate Transition7/1 -> b1/1, [a1]
  Rate Transition/1 -> Simulink-PS Converter/1
  Rate Transition5/1 -> Simulink-PS Converter5/1
  Rate Transition4/1 -> Simulink-PS Converter4/1
  Rate Transition3/1 -> Simulink-PS Converter3/1
  Rate Transition2/1 -> Simulink-PS Converter2/1
  Rate Transition1/1 -> Simulink-PS Converter1/1
  PS-Simulink Converter21/1 -> Rate Transition26/1
  PS-Simulink Converter20/1 -> Rate Transition27/1
  PS-Simulink Converter23/1 -> Rate Transition28/1
  PS-Simulink Converter22/1 -> Rate Transition29/1
  PS-Simulink Converter17/1 -> Rate Transition22/1
  PS-Simulink Converter16/1 -> Rate Transition23/1
  PS-Simulink Converter19/1 -> Rate Transition24/1
  PS-Simulink Converter13/1 -> Rate Transition21/1
  PS-Simulink Converter12/1 -> Rate Transition20/1
  PS-Simulink Converter15/1 -> Rate Transition19/1
  PS-Simulink Converter14/1 -> Rate Transition18/1
  PS-Simulink Converter11/1 -> Rate Transition14/1
  PS-Simulink Converter10/1 -> Rate Transition15/1
  PS-Simulink Converter9/1 -> Rate Transition16/1
  PS-Simulink Converter8/1 -> Rate Transition17/1
  PS-Simulink Converter4/1 -> Rate Transition10/1
  PS-Simulink Converter6/1 -> Rate Transition12/1
  PS-Simulink Converter5/1 -> Rate Transition11/1
  PS-Simulink Converter18/1 -> Rate Transition25/1
  PS-Simulink Converter7/1 -> Rate Transition13/1
  PS-Simulink Converter3/1 -> Rate Transition6/1
  PS-Simulink Converter2/1 -> Rate Transition7/1
  PS-Simulink Converter1/1 -> Rate Transition8/1
  PS-Simulink Converter/1 -> Rate Transition9/1
  connections:
  joint1/LConn2 -- Simulink-PS Converter/RConn1
  joint6/RConn5 -- PS-Simulink Converter21/LConn1
  joint6/RConn4 -- PS-Simulink Converter20/LConn1
  joint6/RConn3 -- PS-Simulink Converter23/LConn1
  joint6/RConn2 -- PS-Simulink Converter22/LConn1
  joint5/RConn5 -- PS-Simulink Converter17/LConn1
  joint5/RConn4 -- PS-Simulink Converter16/LConn1
  joint5/RConn3 -- PS-Simulink Converter19/LConn1
  joint5/RConn2 -- PS-Simulink Converter18/LConn1
  joint4/RConn5 -- PS-Simulink Converter13/LConn1
  joint4/RConn4 -- PS-Simulink Converter12/LConn1
  joint4/RConn3 -- PS-Simulink Converter15/LConn1
  joint4/RConn2 -- PS-Simulink Converter14/LConn1
  joint3/RConn5 -- PS-Simulink Converter11/LConn1
  joint3/RConn4 -- PS-Simulink Converter10/LConn1
  joint3/RConn3 -- PS-Simulink Converter9/LConn1
  joint3/RConn2 -- PS-Simulink Converter8/LConn1
  joint2/RConn5 -- PS-Simulink Converter7/LConn1
  joint2/RConn4 -- PS-Simulink Converter6/LConn1
  joint2/RConn3 -- PS-Simulink Converter5/LConn1
  joint2/RConn2 -- PS-Simulink Converter4/LConn1
  joint1/RConn5 -- PS-Simulink Converter3/LConn1
  PS-Simulink Converter2/LConn1 -- joint1/RConn4
  joint1/RConn3 -- PS-Simulink Converter1/LConn1
  joint1/RConn2 -- PS-Simulink Converter/LConn1
  Simulink-PS Converter5/RConn1 -- joint6/LConn2
  Simulink-PS Converter4/RConn1 -- joint5/LConn2
  Simulink-PS Converter3/RConn1 -- joint4/LConn2
  Simulink-PS Converter2/RConn1 -- joint3/LConn2
  Simulink-PS Converter1/RConn1 -- joint2/LConn2
  World/RConn1 -- Solver Configuration/RConn1 -- Mechanism Configuration/RConn1 -- base/LConn1
  link3/RConn1 -- joint4/LConn1
  link5/LConn1 -- joint5/RConn1
  link4/RConn1 -- joint5/LConn1
  link4/LConn1 -- joint4/RConn1
  link3/LConn1 -- joint3/RConn1
  link2/RConn1 -- joint3/LConn1
  link1/LConn1 -- joint1/RConn1
  base/RConn1 -- joint1/LConn1
  link1/RConn1 -- joint2/LConn1
  link2/LConn1 -- joint2/RConn1
  link5/RConn1 -- joint6/LConn1
  link6/LConn1 -- joint6/RConn1

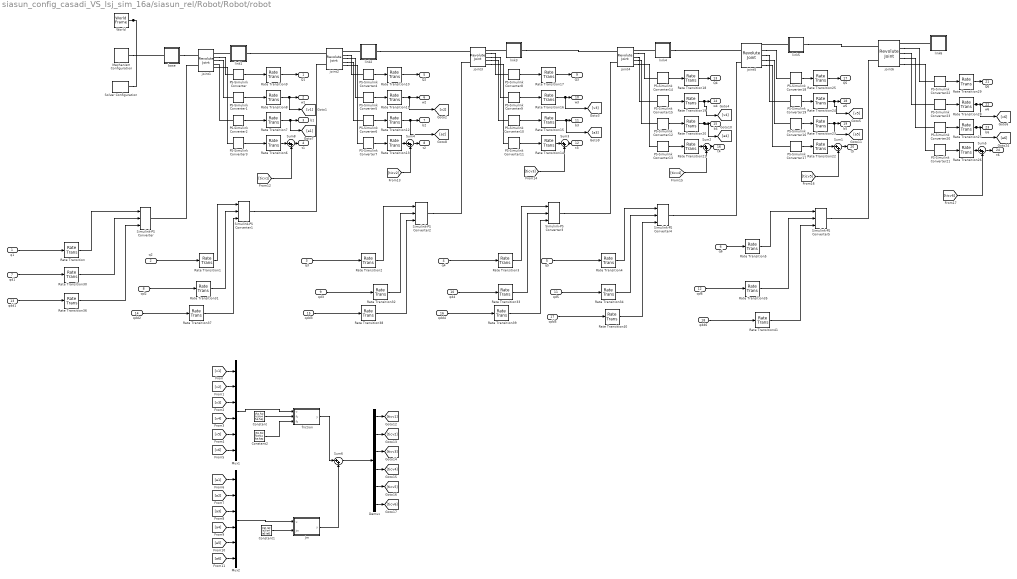
== system siasun_config_casadi_VS_lsj_sim_16a/siasun_rel/Robot/Robot/robot ==
  q1 : Inport
  q2 : Inport  Port=2
  q3 : Inport  Port=3
  q4 : Inport  Port=4
  q5 : Inport  Port=5
  q6 : Inport  Port=6
  qd1 : Inport  Port=7
  qd2 : Inport  Port=8
  qd3 : Inport  Port=9
  qd4 : Inport  Port=10
  qd5 : Inport  Port=11
  qd6 : Inport  Port=12
  qdd1 : Inport  Port=13
  qdd2 : Inport  Port=14
  qdd3 : Inport  Port=15
  qdd4 : Inport  Port=16
  qdd5 : Inport  Port=17
  qdd6 : Inport  Port=18
  Constant : Constant  Value=[fv1 fv2 fv3 fv4 fv5 fv6]
  Constant1 : Constant  Value=[Ia1 Ia2 Ia3 Ia4 Ia5 Ia6]
  Constant2 : Constant  Value=[fc1 fc2 fc3 fc4 fc5 fc6]
  Demux : Demux  Outputs=6
  Jm : MATLAB Function  TreatAsAtomicUnit=on
  Mechanism Configuration : sm_lib/Utilities/Mechanism Configuration  UniformGravity=Constant  GravityVector=[0 0 -9.802]  GravityUnits=m/s^2  LinearizationDelta=0.001
  Mux1 : Mux  Inputs=6
  Mux2 : Mux  Inputs=6
  PS-Simulink Converter{,4,8,14,18,22} (6 alike) : nesl_utility/PS-Simulink Converter  PhysicalDomain=network_engine_domain  SubClassName=ps_output  LeftPortType=input  RightPortType=output  PseudoPeriodic=off  Frequencies=[]  Unit=rad  AffineConversion=off
  PS-Simulink Converter{1,5,9,15,19,23} (6 alike) : nesl_utility/PS-Simulink Converter  PhysicalDomain=network_engine_domain  SubClassName=ps_output  LeftPortType=input  RightPortType=output  PseudoPeriodic=off  Frequencies=[]  Unit=rad/s  AffineConversion=off
  PS-Simulink Converter{2,6,10,12,16,20} (6 alike) : nesl_utility/PS-Simulink Converter  PhysicalDomain=network_engine_domain  SubClassName=ps_output  LeftPortType=input  RightPortType=output  PseudoPeriodic=off  Frequencies=[]  Unit=1  AffineConversion=off
  PS-Simulink Converter{3,7,11,13,17,21} (6 alike) : nesl_utility/PS-Simulink Converter  PhysicalDomain=network_engine_domain  SubClassName=ps_output  LeftPortType=input  RightPortType=output  PseudoPeriodic=off  Frequencies=[]  Unit=N*m  AffineConversion=off
  Rate Transition{,1..41} (42 alike) : RateTransition
  Simulink-PS Converter{,1..5} (6 alike) : nesl_utility/Simulink-PS Converter  PhysicalDomain=network_engine_domain  SubClassName=ps_input  LeftPortType=input  RightPortType=output  PseudoPeriodic=off  Frequencies=[]  NoiseDistribution=none  NoiseParameters=[]  Unit=rad  AffineConversion=off  FilteringAndDerivatives=provide  SimscapeFilterOrder=1  InputFilterTimeConstant=0.001  UdotUserProvided=2
  Solver Configuration : nesl_utility/Solver Configuration  PhysicalDomain=network_engine_domain  SubClassName=solver  LeftPortType=input  RightPortType=generic  Tones=[]  Harmonics=[]  SimulateNoise=off  Profile=off  UseLocalSampling=off  EnableSwitchedLinearOptims=on  FrequencyDomain=off  UseCCode=off  RelTol=0.001  AbsTol=1e-06  MinStep=1e-09  ToWorkspace=off  RevertToSquareIcSolve=off  NumHomotopyIterations=100  PhasorMode=off  PhasorModeNumHarmonics=1  DoDC=off  ResidualTolerance=1e-09  UseLocalSolver=off  LocalSolverChoice=NE_BACKWARD_EULER_ADVANCER  LocalSolverSampleTime=0.001  DoFixedCost=off  MaxNonlinIter=3  MaxModeIter=2  LinearAlgebra=Sparse  EquationFormulation=NE_TIME_EF  DelaysMemoryBudget=1024  AutomaticFiltering=on  FilteringTimeConstant=0.001  PartitionStorageMethod=AS_NEEDED  PartitionMemoryBudget=1024  PartitionMethod=FAST
  Sum{1..6,8} (7 alike) : Sum  Inputs=|++
  World : sm_lib/Frames and Transforms/World Frame
  base : Subsystem
  friction : MATLAB Function  TreatAsAtomicUnit=on
  joint1 : sm_lib/Joints/Revolute Joint  JointMode=Normal  SenseConstraintForce=off  SenseConstraintForceX=off  SenseConstraintForceY=off  SenseConstraintForceZ=off  SenseConstraintTorque=off  SenseConstraintTorqueX=off  SenseConstraintTorqueY=off  SenseConstraintTorqueZ=off  SenseTotalForce=off  SenseTotalForceX=off  SenseTotalForceY=off  SenseTotalForceZ=off  SenseTotalTorque=off  SenseTotalTorqueX=off  SenseTotalTorqueY=off  SenseTotalTorqueZ=off  CompositeWrenchDir=FollowerOnBase  CompositeWrenchFrame=FollowerFrame  EquilibriumPosition=0  EquilibriumPositionUnits=deg  SpringStiffness=0  SpringStiffnessUnits=N*m/deg  DampingCoefficient=0  DampingCoefficientUnits=N*m/(deg/s)  TorqueActuationMode=ComputedTorque  MotionActuationMode=InputMotion  SensePosition=on  SenseVelocity=on  SenseAcceleration=on  SenseTorqueForce=on  SenseLowerLimitTorqueForce=off  SenseUpperLimitTorqueForce=off  LowerLimitSpecify=off  LowerLimitBound=-90  LowerLimitBoundUnits=deg  LowerLimitStiffness=1e4  LowerLimitStiffnessUnits=N*m/deg  LowerLimitDamping=10  LowerLimitDampingUnits=N*m/(deg/s)  LowerLimitTransitionRegionWidth=0.1  LowerLimitTransitionRegionWidthUnits=deg  UpperLimitSpecify=off  UpperLimitBound=90  UpperLimitBoundUnits=deg  UpperLimitStiffness=1e4  UpperLimitStiffnessUnits=N*m/deg  UpperLimitDamping=10  UpperLimitDampingUnits=N*m/(deg/s)  UpperLimitTransitionRegionWidth=0.1  UpperLimitTransitionRegionWidthUnits=deg  PositionTargetSpecify=off  PositionTargetPriority=High  PositionTargetValue=0  PositionTargetValueUnits=deg  VelocityTargetSpecify=off  VelocityTargetPriority=High  VelocityTargetValue=0  VelocityTargetValueUnits=deg/s
  joint{2..6} (5 alike) : sm_lib/Joints/Revolute Joint  JointMode=Normal  SenseConstraintForce=off  SenseConstraintForceX=off  SenseConstraintForceY=off  SenseConstraintForceZ=off  SenseConstraintTorque=off  SenseConstraintTorqueX=off  SenseConstraintTorqueY=off  SenseConstraintTorqueZ=off  SenseTotalForce=off  SenseTotalForceX=off  SenseTotalForceY=off  SenseTotalForceZ=off  SenseTotalTorque=off  SenseTotalTorqueX=off  SenseTotalTorqueY=off  SenseTotalTorqueZ=off  CompositeWrenchDir=FollowerOnBase  CompositeWrenchFrame=BaseFrame  EquilibriumPosition=0  EquilibriumPositionUnits=deg  SpringStiffness=0  SpringStiffnessUnits=N*m/deg  DampingCoefficient=0  DampingCoefficientUnits=N*m/(deg/s)  TorqueActuationMode=ComputedTorque  MotionActuationMode=InputMotion  SensePosition=on  SenseVelocity=on  SenseAcceleration=on  SenseTorqueForce=on  SenseLowerLimitTorqueForce=off  SenseUpperLimitTorqueForce=off  LowerLimitSpecify=off  LowerLimitBound=-90  LowerLimitBoundUnits=deg  LowerLimitStiffness=1e4  LowerLimitStiffnessUnits=N*m/deg  LowerLimitDamping=10  LowerLimitDampingUnits=N*m/(deg/s)  LowerLimitTransitionRegionWidth=0.1  LowerLimitTransitionRegionWidthUnits=deg  UpperLimitSpecify=off  UpperLimitBound=90  UpperLimitBoundUnits=deg  UpperLimitStiffness=1e4  UpperLimitStiffnessUnits=N*m/deg  UpperLimitDamping=10  UpperLimitDampingUnits=N*m/(deg/s)  UpperLimitTransitionRegionWidth=0.1  UpperLimitTransitionRegionWidthUnits=deg  PositionTargetSpecify=off  PositionTargetPriority=High  PositionTargetValue=0  PositionTargetValueUnits=deg  VelocityTargetSpecify=off  VelocityTargetPriority=High  VelocityTargetValue=0  VelocityTargetValueUnits=deg/s
  link1 : Subsystem
  link2 : Subsystem
  link3 : Subsystem
  link4 : Subsystem
  link5 : Subsystem
  link6 : Subsystem
  Q1 : Outport
  w1 : Outport  Port=2
  b1 : Outport  Port=3
  t1 : Outport  Port=4
  Q2 : Outport  Port=5
  w2 : Outport  Port=6
  b2 : Outport  Port=7
  t2 : Outport  Port=8
  Q3 : Outport  Port=9
  w3 : Outport  Port=10
  b3 : Outport  Port=11
  t3 : Outport  Port=12
  Q4 : Outport  Port=13
  w4 : Outport  Port=14
  b4 : Outport  Port=15
  t4 : Outport  Port=16
  Q5 : Outport  Port=17
  w5 : Outport  Port=18
  b5 : Outport  Port=19
  t5 : Outport  Port=20
  Q6 : Outport  Port=21
  w6 : Outport  Port=22
  b6 : Outport  Port=23
  t6 : Outport  Port=24
  wires:
  Rate Transition41/1 -> Simulink-PS Converter5/3
  qdd6/1 -> Rate Transition41/1
  Rate Transition40/1 -> Simulink-PS Converter4/3
  qdd5/1 -> Rate Transition40/1
  Rate Transition39/1 -> Simulink-PS Converter3/3
  qdd4/1 -> Rate Transition39/1
  Rate Transition38/1 -> Simulink-PS Converter2/3
  qdd3/1 -> Rate Transition38/1
  Rate Transition37/1 -> Simulink-PS Converter1/3
  qdd2/1 -> Rate Transition37/1
  Rate Transition36/1 -> Simulink-PS Converter/3
  qdd1/1 -> Rate Transition36/1
  Rate Transition35/1 -> Simulink-PS Converter5/2
  qd6/1 -> Rate Transition35/1
  Rate Transition34/1 -> Simulink-PS Converter4/2
  qd5/1 -> Rate Transition34/1
  Rate Transition33/1 -> Simulink-PS Converter3/2
  qd4/1 -> Rate Transition33/1
  Rate Transition32/1 -> Simulink-PS Converter2/2
  qd3/1 -> Rate Transition32/1
  Rate Transition31/1 -> Simulink-PS Converter1/2
  qd2/1 -> Rate Transition31/1
  Rate Transition30/1 -> Simulink-PS Converter/2
  qd1/1 -> Rate Transition30/1
  Rate Transition6/1 -> Sum8/1
  Sum8/1 -> t1/1
  [ticv2] -> Sum4/2
  Sum4/1 -> t2/1
  Rate Transition13/1 -> Sum4/1
  Sum3/1 -> t3/1
  Rate Transition14/1 -> Sum3/1
  Sum2/1 -> t4/1
  Rate Transition21/1 -> Sum2/1
  Sum1/1 -> t5/1
  Rate Transition22/1 -> Sum1/1
  Sum5/1 -> t6/1
  Rate Transition26/1 -> Sum5/1
  q6/1 -> Rate Transition5/1
  q5/1 -> Rate Transition4/1
  q4/1 -> Rate Transition3/1
  q3/1 -> Rate Transition2/1
  q2/1 -> Rate Transition1/1
  q1/1 -> Rate Transition/1
  Sum6/1 -> Demux/1
  Constant2/1 -> friction/3(fc)
  Constant1/1 -> Jm/2(Jm)
  Constant/1 -> friction/2(fv)
  Jm/1(y) -> Sum6/2
  friction/1(y) -> Sum6/1
  Mux2/1 -> Jm/1(u)
  Mux1/1 -> friction/1(u)
  [ticv6] -> Sum5/2
  [ticv5] -> Sum1/2
  [ticv4] -> Sum2/2
  [ticv3] -> Sum3/2
  [ticv1] -> Sum8/2
  Demux/6 -> [ticv6]
  Demux/5 -> [ticv5]
  Demux/4 -> [ticv4]
  Demux/3 -> [ticv3]
  Demux/2 -> [ticv2]
  Demux/1 -> [ticv1]
  [a6] -> Mux2/6
  [a4] -> Mux2/4
  [a5] -> Mux2/5
  [a3] -> Mux2/3
  [a2] -> Mux2/2
  [a1] -> Mux2/1
  [v6] -> Mux1/6
  [v5] -> Mux1/5
  [v4] -> Mux1/4
  [v3] -> Mux1/3
  [v2] -> Mux1/2
  [v1] -> Mux1/1
  Rate Transition29/1 -> Q6/1
  Rate Transition28/1 -> w6/1, [v6]
  Rate Transition27/1 -> b6/1, [a6]
  Rate Transition25/1 -> Q5/1
  Rate Transition24/1 -> w5/1, [v5]
  Rate Transition23/1 -> b5/1, [a5]
  Rate Transition20/1 -> b4/1, [a4]
  Rate Transition19/1 -> w4/1, [v4]
  Rate Transition18/1 -> Q4/1
  Rate Transition17/1 -> Q3/1
  Rate Transition16/1 -> w3/1, [v3]
  Rate Transition15/1 -> b3/1, [a3]
  Rate Transition12/1 -> b2/1, [a2]
  Rate Transition11/1 -> w2/1, [v2]
  Rate Transition10/1 -> Q2/1
  Rate Transition9/1 -> Q1/1
  Rate Transition8/1 -> w1/1, [v1]
  Rate Transition7/1 -> b1/1, [a1]
  Rate Transition/1 -> Simulink-PS Converter/1
  Rate Transition5/1 -> Simulink-PS Converter5/1
  Rate Transition4/1 -> Simulink-PS Converter4/1
  Rate Transition3/1 -> Simulink-PS Converter3/1
  Rate Transition2/1 -> Simulink-PS Converter2/1
  Rate Transition1/1 -> Simulink-PS Converter1/1
  PS-Simulink Converter21/1 -> Rate Transition26/1
  PS-Simulink Converter20/1 -> Rate Transition27/1
  PS-Simulink Converter23/1 -> Rate Transition28/1
  PS-Simulink Converter22/1 -> Rate Transition29/1
  PS-Simulink Converter17/1 -> Rate Transition22/1
  PS-Simulink Converter16/1 -> Rate Transition23/1
  PS-Simulink Converter19/1 -> Rate Transition24/1
  PS-Simulink Converter13/1 -> Rate Transition21/1
  PS-Simulink Converter12/1 -> Rate Transition20/1
  PS-Simulink Converter15/1 -> Rate Transition19/1
  PS-Simulink Converter14/1 -> Rate Transition18/1
  PS-Simulink Converter11/1 -> Rate Transition14/1
  PS-Simulink Converter10/1 -> Rate Transition15/1
  PS-Simulink Converter9/1 -> Rate Transition16/1
  PS-Simulink Converter8/1 -> Rate Transition17/1
  PS-Simulink Converter4/1 -> Rate Transition10/1
  PS-Simulink Converter6/1 -> Rate Transition12/1
  PS-Simulink Converter5/1 -> Rate Transition11/1
  PS-Simulink Converter18/1 -> Rate Transition25/1
  PS-Simulink Converter7/1 -> Rate Transition13/1
  PS-Simulink Converter3/1 -> Rate Transition6/1
  PS-Simulink Converter2/1 -> Rate Transition7/1
  PS-Simulink Converter1/1 -> Rate Transition8/1
  PS-Simulink Converter/1 -> Rate Transition9/1
  connections:
  joint1/LConn2 -- Simulink-PS Converter/RConn1
  joint6/RConn5 -- PS-Simulink Converter21/LConn1
  joint6/RConn4 -- PS-Simulink Converter20/LConn1
  joint6/RConn3 -- PS-Simulink Converter23/LConn1
  joint6/RConn2 -- PS-Simulink Converter22/LConn1
  joint5/RConn5 -- PS-Simulink Converter17/LConn1
  joint5/RConn4 -- PS-Simulink Converter16/LConn1
  joint5/RConn3 -- PS-Simulink Converter19/LConn1
  joint5/RConn2 -- PS-Simulink Converter18/LConn1
  joint4/RConn5 -- PS-Simulink Converter13/LConn1
  joint4/RConn4 -- PS-Simulink Converter12/LConn1
  joint4/RConn3 -- PS-Simulink Converter15/LConn1
  joint4/RConn2 -- PS-Simulink Converter14/LConn1
  joint3/RConn5 -- PS-Simulink Converter11/LConn1
  joint3/RConn4 -- PS-Simulink Converter10/LConn1
  joint3/RConn3 -- PS-Simulink Converter9/LConn1
  joint3/RConn2 -- PS-Simulink Converter8/LConn1
  joint2/RConn5 -- PS-Simulink Converter7/LConn1
  joint2/RConn4 -- PS-Simulink Converter6/LConn1
  joint2/RConn3 -- PS-Simulink Converter5/LConn1
  joint2/RConn2 -- PS-Simulink Converter4/LConn1
  joint1/RConn5 -- PS-Simulink Converter3/LConn1
  PS-Simulink Converter2/LConn1 -- joint1/RConn4
  joint1/RConn3 -- PS-Simulink Converter1/LConn1
  joint1/RConn2 -- PS-Simulink Converter/LConn1
  Simulink-PS Converter5/RConn1 -- joint6/LConn2
  Simulink-PS Converter4/RConn1 -- joint5/LConn2
  Simulink-PS Converter3/RConn1 -- joint4/LConn2
  Simulink-PS Converter2/RConn1 -- joint3/LConn2
  Simulink-PS Converter1/RConn1 -- joint2/LConn2
  World/RConn1 -- Solver Configuration/RConn1 -- Mechanism Configuration/RConn1 -- base/LConn1
  link3/RConn1 -- joint4/LConn1
  link5/LConn1 -- joint5/RConn1
  link4/RConn1 -- joint5/LConn1
  link4/LConn1 -- joint4/RConn1
  link3/LConn1 -- joint3/RConn1
  link2/RConn1 -- joint3/LConn1
  link1/LConn1 -- joint1/RConn1
  base/RConn1 -- joint1/LConn1
  link1/RConn1 -- joint2/LConn1
  link2/LConn1 -- joint2/RConn1
  link5/RConn1 -- joint6/LConn1
  link6/LConn1 -- joint6/RConn1
